simulink model "Federpendelmodell"  (R2014a)
settings: Solver=ode45  StartTime=0.0  StopTime=4.5  RelTol=1e-3
InitFcn:
  | % Parameter laden
  | Parameter_Aufgabe_3_1;
values from neighbouring files (symbols this model uses):
  c = 10    [Parameter_Aufgabe_3_1.m]
  d = 0.5    [Parameter_Aufgabe_3_1.m]
  g = 9.81    [Parameter_Aufgabe_3_1.m]
  m = 0.2    [Parameter_Aufgabe_3_1.m]
libraries: simulink x1
settings Model: Creator=Glöckler  LastModifiedBy=Glöckler
settings OptimizationCC: ExpressionDepthLimit=2147483647
settings DebuggingCC: UnderspecifiedInitializationDetection=Classic  StateNameClashWarn=warning

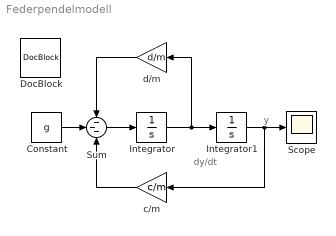
== system Federpendelmodell ==
  note: y
  note: dy/dt
  Constant : Constant  Value=g
  DocBlock : simulink/Model-Wide Utilities/DocBlock  DocumentType=Text
      content=|
      | % Parameter:
      | m = 0.2;    % Masse [kg]
      | c = 10;     % Federsteifigkeit [N/m]
      | d = 0.5;    % Dämpfungskonstante [Ns/m]
      | g = 9.81;   % Erdbeschleunigung
      |
      | % Die Parameter werden automatisch vor dem Start der Simulation geladen.
      | % Siehe: File/Model Properties/Callbacks/InitFcn
      | %
  Integrator : Integrator
  Integrator1 : Integrator
  Scope : Scope
      settings: TimeRange=5  YMin=-0.35  YMax=0
  Sum : Sum  Inputs=---
  c/m : Gain  Gain=c/m
  d/m : Gain  Gain=d/m
  wires:
  Sum/1 -> Integrator/1
  Integrator/1 -> Integrator1/1, d/m/1
  Integrator1/1 -> Scope/1, c/m/1
  Constant/1 -> Sum/2
  d/m/1 -> Sum/1
  c/m/1 -> Sum/3
